simulink model "untitled"  (Simulink 6.6)
settings: Solver=ode3  StartTime=0.0  StopTime=0.2  FixedStep=0.001  RelTol=1e-3
settings Model: Creator=student  LastModifiedBy=student

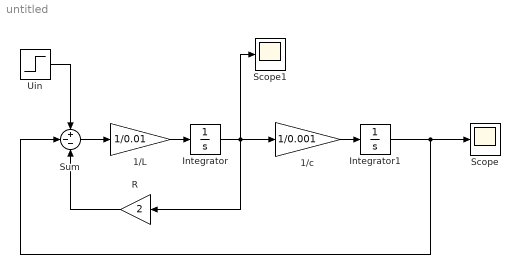
== system untitled ==
  1/L : Gain  Gain=1/0.01
  1/c : Gain  Gain=1/0.001
  Integrator : Integrator  InitialCondition=1
  Integrator1 : Integrator
  R : Gain  Orientation=left  Gain=2
  Scope : Scope
  Scope1 : Scope
      settings: TimeRange=5
  Sum : Sum  Inputs=+--
  Uin : Step  Time=0.1  After=5  SampleTime=0
  wires:
  Sum/1 -> 1/L/1
  1/L/1 -> Integrator/1
  Integrator/1 -> 1/c/1, R/1, Scope1/1
  1/c/1 -> Integrator1/1
  Integrator1/1 -> Scope/1, Sum/2
  R/1 -> Sum/3
  Uin/1 -> Sum/1
